simulink model "slexIonosphereClassificationTreePredictExample"  (R2023a)
settings: Solver=FixedStepDiscrete  StartTime=0.0  StopTime=radarReturnInput.time(end)  RelTol=1e-3
PreLoadFcn:
  | if ~exist("treeMdl","var")
  | 
  | load ionosphere
  | 
  | prsntX = X(1:300,:);
  | prsntY = Y(1:300);
  | ftrX = X(301:end,:);
  | ftrY = Y(301:end);
  | 
  | trainedModel = trainClassificationTreeModel(prsntX,prsntY);
  | treeMdl = trainedModel.ClassificationTree;
  | 
  | radarReturnInput.time = (0:50)';
  | radarReturnInput.signals(1).values = ftrX;
  | radarReturnInput.signals(1).dimensions = size(ftrX,2);
  | 
  | end
libraries: statsLibrary x1
settings Model: Creator=The MathWorks, Inc.  LastModifiedBy=The MathWorks, Inc.
settings SolverCC: AlgebraicLoopSolver=TrustRegion
settings DataIOCC: ExternalInput=radarReturnInput  LoadExternalInput=on
settings DebuggingCC: UnconnectedInputMsg=warning  UnconnectedOutputMsg=warning  UnconnectedLineMsg=warning
settings ModelReferenceCC: EnableRefExpFcnMdlSchedulingChecks=on
settings RTWCC: DLArmComputeVersion=19.05

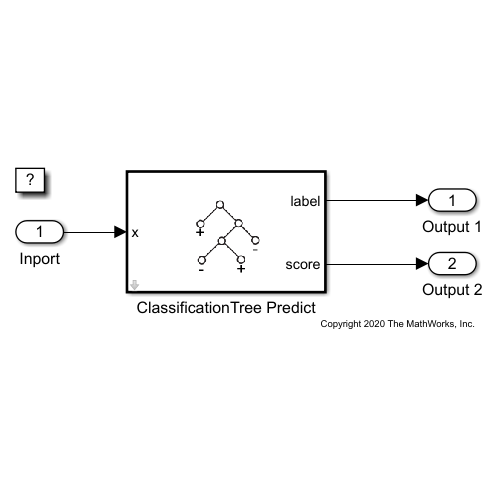
[thumbnail: Simulink's stored preview of the top-level diagram]
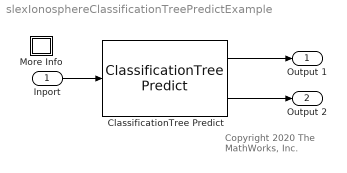
== system slexIonosphereClassificationTreePredictExample ==
  note: Copyright 2020 The MathWorks, Inc.
  Inport : Inport  PortDimensions=34
  ClassificationTree Predict : statsLibrary/Classification/ClassificationTree Predict  TrainedLearner=treeMdl  ShowOutputScore=on  LabelOutMin=[]  LabelOutMax=[]  ScoreOutMin=[]  ScoreOutMax=[]  RawScoreOutMin=[]  RawScoreOutMax=[]  StoredEnumName=treeMdl_enumLabels
  More Info : Subsystem
      settings: OpenFcn=showExample('stats/PredictClassLabelsUsingClassificationTreePredictBlockExample')
      mask Display: disp('?')
  Output 1 : Outport
  Output 2 : Outport  Port=2
  wires:
  Inport/1 -> ClassificationTree Predict/1
  ClassificationTree Predict/1 -> Output 1/1
  ClassificationTree Predict/2 -> Output 2/1

== system slexIonosphereClassificationTreePredictExample/More Info ==
